simulink model "MATLAB_Exercise_6A"  (R2017b)
settings: Solver=VariableStepAuto  StartTime=0.0  StopTime=1  FixedStep=0.0001  RelTol=1e-3
settings Model: Creator=chenjiasheng  LastModifiedBy=chenjiasheng

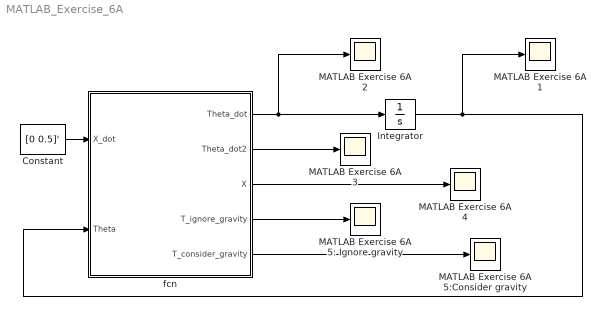
== system MATLAB_Exercise_6A ==
  Constant : Constant  Value=[0 0.5]'
  Integrator : Integrator  InitialCondition=[pi/18 pi/2]'
  MATLAB Exercise 6A {1..4} (4 alike) : Scope
  MATLAB Exercise 6A 5: Ignore gravity : Scope
  MATLAB Exercise 6A 5:Consider gravity : Scope
  fcn : MATLAB Function  TreatAsAtomicUnit=on
  wires:
  fcn/1(Theta_dot) -> MATLAB Exercise 6A 2/1, Integrator/1
  Integrator/1 -> fcn/2(Theta), MATLAB Exercise 6A 1/1
  Constant/1 -> fcn/1(X_dot)
  fcn/3(X) -> MATLAB Exercise 6A 4/1
  fcn/2(Theta_dot2) -> MATLAB Exercise 6A 3/1
  fcn/4(T_ignore_gravity) -> MATLAB Exercise 6A 5: Ignore gravity/1
  fcn/5(T_consider_gravity) -> MATLAB Exercise 6A 5:Consider gravity/1

== matlab function MATLAB_Exercise_6A/fcn ==
  data: X_dot input; Theta_dot output; Theta_dot2 output; Theta input; X output; T_ignore_gravity output; T_consider_gravity output
function [Theta_dot,Theta_dot2,X,T_ignore_gravity,T_consider_gravity] = fcn(X_dot,Theta)
L1=1;
L2=0.5;
w=0.05;
t=0.05;
m1=19.515;
m2=9.7575;
g=9.81;
I1=[m1/12*(w^2+t^2) 0                0;
    0               m1/12*(L1^2+t^2) 0;
    0               0                m1/12*(L1^2+w^2)];
I2=[m2/12*(w^2+t^2) 0                0;
    0               m2/12*(L2^2+t^2) 0;
    0               0                m2/12*(L2^2+w^2)];
%--------------------------
theta1=Theta(1)
theta2=Theta(2)
J=[-L1*sin(theta1)-L2*sin(theta1+theta2) -L2*sin(theta1+theta2);
    L1*cos(theta1)+L2*cos(theta1+theta2)  L2*cos(theta1+theta2)];
Theta_dot=inv(J)*X_dot;
theta1_dot=Theta_dot(1);
theta2_dot=Theta_dot(2);
%------------------------
J_dot=[-L1*cos(theta1)*theta1_dot-L2*cos(theta1+theta2)*(theta1_dot+theta2_dot) -L2*cos(theta1+theta2)*(theta1_dot+theta2_dot);
       -L1*sin(theta1)*theta1_dot-L2*sin(theta1+theta2)*(theta1_dot+theta2_dot) -L2*sin(theta1+theta2)*(theta1_dot+theta2_dot)]
Theta_dot2=-inv(J)*J_dot*Theta_dot;
theta1_dot2=Theta_dot2(1);
theta2_dot2=Theta_dot2(2);
%------------------------
x=L1*cos(theta1)+L2*cos(theta1+theta2);
y=L1*sin(theta1)+L2*sin(theta1+theta2);
phi=theta1+theta2;
X=[x y phi]'
%-------------------------
% ignore gravity
omega1=[0 0 theta1_dot]';
omega1_dot=[0 0 theta1_dot2]';
vC1_dot=[-L1/2*theta1_dot^2, L1/2*theta1_dot2, 0]';
F1=m1*vC1_dot;
N1=I1*omega1_dot+cross(omega1,I1*omega1);
omega2=[0 0 theta1_dot+theta2_dot]';
omega2_dot=[0 0 theta1_dot2+theta2_dot2]';
vC2_dot=[-L1*theta1_dot^2*cos(theta2)+L1*theta1_dot2*sin(theta2)-L2/2*(theta1_dot+theta2_dot)^2;
          L1*theta1_dot^2*sin(theta2)+L1*theta1_dot2*cos(theta2)+L2/2*(theta1_dot2+theta2_dot2);
          0];
F2=m2*vC2_dot
N2=I2*omega2_dot+cross(omega2,I2*omega2)
f2=F2
n2=N2+cross([L2/2 0 0]',F2)
tau2=n2'*[0 0 1]'
R12=[cos(theta2) -sin(theta2) 0;
     sin(theta2)  cos(theta2) 0;
     0            0           1];
f1=R12*f2+F1
n1=N1+R12*n2+cross([L1/2 0 0]',F1)+cross([L1 0 0]',R12*f2)
tau1=n1'*[0 0 1]'
T_ignore_gravity=[tau1 tau2]'
%-------------------------------------
% consider gravity
omega1=[0 0 theta1_dot]';
omega1_dot=[0 0 theta1_dot2]';
vC1_dot=[-L1/2*theta1_dot^2+g*sin(theta1), L1/2*theta1_dot2+g*cos(theta1), 0]';
F1=m1*vC1_dot;
N1=I1*omega1_dot+cross(omega1,I1*omega1);
omega2=[0 0 theta1_dot+theta2_dot]';
omega2_dot=[0 0 theta1_dot2+theta2_dot2]';
vC2_dot=[-L1*theta1_dot^2*cos(theta2)+L1*theta1_dot2*sin(theta2)+g*sin(theta1+theta2)-L2/2*(theta1_dot+theta2_dot)^2;
          L1*theta1_dot^2*sin(theta2)+L1*theta1_dot2*cos(theta2)+g*cos(theta1+theta2)+L2/2*(theta1_dot2+theta2_dot2);
          0];
F2=m2*vC2_dot
N2=I2*omega2_dot+cross(omega2,I2*omega2)
f2=F2
n2=N2+cross([L2/2 0 0]',F2)
tau2=n2'*[0 0 1]'
R12=[cos(theta2) -sin(theta2) 0;
     sin(theta2)  cos(theta2) 0;
     0            0           1];
f1=R12*f2+F1
n1=N1+R12*n2+cross([L1/2 0 0]',F1)+cross([L1 0 0]',R12*f2)
tau1=n1'*[0 0 1]'
T_consider_gravity=[tau1 tau2]'
end
